simulink model "AcermanDynExt"  (R2019b)
settings: Solver=FixedStepAuto  StartTime=0.0  StopTime=simTime  RelTol=1e-3
values from neighbouring files (symbols this model uses):
  a0 = 1    [Ackerman_init.m]
  a1 = 4    [Ackerman_init.m]
  a2 = 3    [Ackerman_init.m]
  Change = 0    [Ackerman_init.m]
  k0 = 1    [Ackerman_init.m]
  k1 = place(Ad,bd,pd)    [Ackerman_init.m]
  k2 = place(Ac,bc,lambdatr')    [Ackerman_init.m]
  l = ylabel('$\omega(t)$' )    [Ackerman_init.m]
  pathType = 1    [Ackerman_init.m]
  phi0 = 0    [Ackerman_init.m]
  r = 2    [Ackerman_init.m]
  ref0 = [0 0]'    [Ackerman_init.m]
  refType = 1    [Ackerman_init.m]
  T = 0.324    [Ackerman_init.m]
  theta0 = pi/2    (= 1.57079632679)    [Ackerman_init.m]
  v0 = 1    [Ackerman_init.m]
  v_ref = 2    [Ackerman_init.m]
  x0 = 1    [Ackerman_init.m]
  y0 = 1    [Ackerman_init.m]
libraries: robotmobilelib x5
(part 4 of 6)

== matlab function AcermanDynExt/MATLAB Function6 ==
  data: c_old input; c output
function c  = fcn(c_old)

if c_old < 3
    c = c_old+1; 
else 
    c = 0;  
end

== matlab function AcermanDynExt/MATLAB Function7 ==
  data: ref_old input; delta_b input; ref_x1 output; v0 input; ref_x output; m parameter
function [ref_x1,ref_x] = fcn(ref_old, delta_b, v0, m)
delta = delta_b*3; 
a1 = m;
ref_old(2) = 0; 

ref_x1 = ref_old + [delta*v0*a1; v0*a1];

ref_x2 = ref_x1 + [delta*v0*a1; v0*a1];
ref_x = [ref_x1 ref_x2];

== matlab function AcermanDynExt/MATLAB Function8 ==
  data: tnref input; ref output; refType parameter; v_ref parameter
function ref = fcn(tnref,refType,v_ref)

if (refType == 1)
    ref = v_ref;
else
    ref = tnref(1,2);
    
end

== matlab function AcermanDynExt/MATLAB Function10 ==
  data: state input; v input; vsdd input; v_ref input; pathType parameter; r parameter; k0 parameter; l parameter; utn output; utr output; Change parameter; T parameter; refType parameter; k1 parameter
function [utn,utr] = MATLAB_Function5(state, v, vsdd, v_ref,pathType, r, k0, l , Change, T, refType, k1)

x = state(1); y = state(2); theta = state(3); phi = state(4);
eta1 = v; eta2 = vsdd;

if pathType == 1
    D = [ -(y*cos(theta) - x*sin(theta))/(x^2 + y^2), (eta1^2*(x*cos(theta) + y*sin(theta)))/(l*cos(phi)^2*(x^2 + y^2));
            2*x*cos(theta) + 2*y*sin(theta),           (2*eta1^2*(y*cos(theta) - x*sin(theta)))/(l*cos(phi)^2)];
    F  = [  (eta1*(sin(phi)*x^2 - 2*l*cos(phi)*sin(theta)*x + sin(phi)*y^2 + 2*l*cos(phi)*cos(theta)*y)*(eta1^2*l*x^2*cos(phi) - 3*eta1^2*l*y^2*cos(phi) + eta1^2*y^3*cos(theta)*sin(phi) - eta1^2*x^3*sin(phi)*sin(theta) + eta1^2*x^2*y*cos(theta)*sin(phi) - eta1^2*x*y^2*sin(phi)*sin(theta) - 4*eta1^2*l*x^2*cos(phi)*cos(theta)^2 + 4*eta1^2*l*y^2*cos(phi)*cos(theta)^2 + 3*eta2*l*x^3*cos(phi)*cos(theta) + 3*eta2*l*y^3*cos(phi)*sin(theta) + 3*eta2*l*x*y^2*cos(phi)*cos(theta) + 3*eta2*l*x^2*y*cos(phi)*sin(theta) - 8*eta1^2*l*x*y*cos(phi)*cos(theta)*sin(theta)))/(l^2*cos(phi)^2*(x^2 + y^2)^3);
                                                                                                                                                                                                                                                                                                                                           (2*eta1*(3*eta2*l^2*cos(phi)^2*sin(theta)^2 - eta1^2*x*cos(theta)*sin(phi)^2 - eta1^2*y*sin(phi)^2*sin(theta) + 3*eta2*l^2*cos(phi)^2*cos(theta)^2 + 3*eta2*l*y*cos(phi)*cos(theta)*sin(phi) - 3*eta2*l*x*cos(phi)*sin(phi)*sin(theta)))/(l^2*cos(phi)^2)];
else

    D = [ -(y*cos(theta)-x*sin(theta))/(x^2 + y^2),  (eta1^2*(x*cos(theta)+y*sin(theta)))/(cos(phi)^2*(x^2+y^2));
         4*x*cos(theta)*(x^2 + y^2-9)+4*y*sin(theta)*(x^2 + y^2+9),    eta1*(tan(phi)^2+1)*(4*y*eta1*cos(theta)*(x^2 + y^2+9)-4*x*eta1*sin(theta)*(x^2 + y^2-9))];
 
     F  = [ (eta1*(sin(phi)*x^2-2*cos(phi)*sin(theta)*x+sin(phi)*y^2+2*cos(theta)*cos(phi)*y)*(x^2*eta1^2*cos(phi)-3*y^2*eta1^2*cos(phi)-4*x^2*eta1^2*cos(theta)^2*cos(phi)+4*y^2*eta1^2*cos(theta)^2*cos(phi)+3*x^3*eta2*cos(theta)*cos(phi)+3*y^3*eta2*cos(phi)*sin(theta)+y^3*eta1^2*cos(theta)*sin(phi)-x^3*eta1^2*sin(theta)*sin(phi)+x^2*y*eta1^2*cos(theta)*sin(phi)-x*y^2*eta1^2*sin(theta)*sin(phi)+3*x*y^2*eta2*cos(theta)*cos(phi)+3*x^2*y*eta2*cos(phi)*sin(theta)-8*x*y*eta1^2*cos(theta)*cos(phi)*sin(theta)))/(cos(phi)^2*(x^2 + y^2)^3);
       (36*x*eta1^3*cos(theta) + 108*eta1*eta2*cos(phi)^2 - 36*y*eta1^3*sin(theta) - 4*x^3*eta1^3*cos(theta) - 4*y^3*eta1^3*sin(theta) + 4*x^3*eta1^3*cos(theta)*cos(phi)^2 + 4*y^3*eta1^3*cos(phi)^2*sin(theta) - 4*x*y^2*eta1^3*cos(theta) + 12*x^2*eta1*eta2*cos(phi)^2 + 36*y^2*eta1*eta2*cos(phi)^2 - 12*x*y*eta1^3*sin(2*phi) - 4*x^2*y*eta1^3*sin(theta) - 12*x*eta1^3*cos(theta)*cos(phi)^2 - 216*eta1*eta2*cos(theta)^2*cos(phi)^2 + 60*y*eta1^3*cos(phi)^2*sin(theta) + 4*x*y^2*eta1^3*cos(theta)*cos(phi)^2 + 24*x^2*eta1*eta2*cos(theta)^2*cos(phi)^2 - 24*y^2*eta1*eta2*cos(theta)^2*cos(phi)^2 + 4*x^2*y*eta1^3*cos(phi)^2*sin(theta) + 216*eta1^3*cos(theta)*cos(phi)*sin(theta)*sin(phi) + 48*x*y*eta1^3*cos(theta)^2*cos(phi)*sin(phi) + 108*y*eta1*eta2*cos(theta)*cos(phi)*sin(phi) + 108*x*eta1*eta2*cos(phi)*sin(theta)*sin(phi) - 24*x^2*eta1^3*cos(theta)*cos(phi)*sin(theta)*sin(phi) + 24*y^2*eta1^3*cos(theta)*cos(phi)*sin(theta)*sin(phi) + 12*y^3*eta1*eta2*cos(theta)*cos(phi)*sin(phi) - 12*x^3*eta1*eta2*cos(phi)*sin(theta)*sin(phi) + 48*x*y*eta1*eta2*cos(theta)*cos(phi)^2*sin(theta) + 12*x^2*y*eta1*eta2*cos(theta)*cos(phi)*sin(phi) - 12*x*y^2*eta1*eta2*cos(phi)*sin(theta)*sin(phi))/cos(phi)^2];
    
end

  
Di = pinv(D);

if pathType == 1
    alpha = x^2+y^2 - r^2;
    psi1 = x^2+y^2-r^2; %
    psi2 = 2*eta1*(x*cos(theta) + y*sin(theta));
    psi3 = 2*eta1^2*cos(theta)^2 + 2*eta1^2*sin(theta)^2 + eta2*(2*x*cos(theta) + 2*y*sin(theta)) + (2*eta1^2*tan(phi)*(y*cos(theta) - x*sin(theta)))/l;

else
    a       = 3; b       = 1.05*a;
    alpha = (x^2+y^2+a^2)^2-4*a^2*x^2-b^4; % defines the path
    psi1 = (x^2+y^2+a^2)^2-4*a^2*x^2-b^4;
    psi2 = 4*x*eta1*cos(theta)*(x^2 + y^2 - 9) + 4*y*eta1*sin(theta)*(x^2 + y^2 + 9);
    psi3 = eta2*(4*x*cos(theta)*(x^2 + y^2 - 9) + 4*y*sin(theta)*(x^2 + y^2 + 9)) + eta1*cos(theta)*(8*x^2*eta1*cos(theta) + 4*eta1*cos(theta)*(x^2 + y^2 - 9) + 8*x*y*eta1*sin(theta)) + eta1*sin(theta)*(8*y^2*eta1*sin(theta) + 4*eta1*sin(theta)*(x^2 + y^2 + 9) + 8*x*y*eta1*cos(theta)) + eta1*tan(phi)*(4*y*eta1*cos(theta)*(x^2 + y^2 + 9) - 4*x*eta1*sin(theta)*(x^2 + y^2 - 9));
end

if alpha < 1e-2 && Change == 1
    ref = 2*v_ref;
else
    ref = v_ref;
end

delta = T;
psi = [psi1-delta*psi2+delta^2/3*psi3;psi2-delta*psi3;psi3];
usd1 = -k0*(eta1-ref)-k0*eta2;
usd2 =  k1*psi;

u  = Di*([usd1;usd2]-F);
utn = u(1); 
utr = u(2);

== matlab function AcermanDynExt/MATLAB Function9 ==
  data: x output; state input; y output; theta output
function [x, y, theta] = fcn(state)

x = state(1);
y = state(2);
theta = state(3);

== matlab function AcermanDynExt/MATLAB Function11 ==
  data: x output; state input; y output; theta output
function [x, y, theta] = fcn(state)

x = state(1);
y = state(2);
theta = state(3);
